simulink model "math_int_2_test"  (Simulink 8.7)
settings: Solver=VariableStepDiscrete  StartTime=0.0  StopTime=10.0  RelTol=1e-3
settings Model: Creator=arnaud  LastModifiedBy=hamza
settings DataIOCC: SaveFormat=Structure  SignalLoggingSaveFormat=ModelDataLogs
settings OptimizationCC: ExpressionDepthLimit=2147483647
settings DebuggingCC: SolverPrmCheckMsg=warning  FcnCallInpInsideContextMsg=UseLocalSettings  StateNameClashWarn=warning  StrictBusMsg=Warning
settings GRTTargetCC: CombineOutputUpdateFcns=off  GRTInterface=on
settings ConfigComp: CovSFcnEnable=off

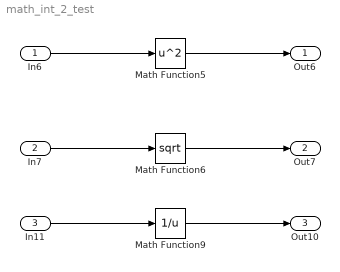
== system math_int_2_test ==
  In6 : Inport  OutDataTypeStr=int32
  In7 : Inport  Port=2  OutDataTypeStr=int8
  In11 : Inport  Port=3  OutDataTypeStr=int8
  Math Function5 : Math  Operator=square  SaturateOnIntegerOverflow=on
  Math Function6 : Math  Operator=sqrt  SaturateOnIntegerOverflow=on
  Math Function9 : Math  Operator=reciprocal  SaturateOnIntegerOverflow=on
  Out6 : Outport
  Out7 : Outport  Port=2
  Out10 : Outport  Port=3
  wires:
  In6/1 -> Math Function5/1
  Math Function5/1 -> Out6/1
  In7/1 -> Math Function6/1
  Math Function6/1 -> Out7/1
  In11/1 -> Math Function9/1
  Math Function9/1 -> Out10/1
